simulink model "c6711dsktest"  (Simulink 6.0)
settings: Solver=FixedStepDiscrete  SolverMode=SingleTasking  StartTime=0.0  StopTime=inf  RelTol=1e-3
libraries: c6711dsklib x3, c6000tgtpreflib x1, dspsrcs4 x1
settings Model: Creator=tjones  LastModifiedBy=thartley  ExtModeTrigMode=oneshot  ExtModeArmWhenConnect=off  ProdHWDeviceType=TI C6000
settings DataIOCC: LimitDataPoints=off  SaveOutput=off  SaveTime=off  SignalLoggingName=sigsOut
settings OptimizationCC: BlockReduction=off  BooleanDataType=off  InlineParams=on  LocalBlockOutputs=off  RollThreshold=2
settings DebuggingCC: AlgebraicLoopMsg=error  CheckExecutionContextPreStartOutputMsg=on  CheckExecutionContextRuntimeOutputMsg=on  SolverPrmCheckMsg=none
settings HardwareCC: ProdBitPerLong=40  ProdEndianess=LittleEndian  ProdHWDeviceType=TI C6000
settings ModelReferenceCC: UpdateModelReferenceTargets=IfOutOfDate
settings RTWCC: SystemTargetFile=ti_c6000.tlc  TemplateMakefile=ti_c6000.tmf  ProcessScript=ti_c6000_make_rtw_hook
settings CodeAppCC: PrefixModelToSubsysFcnNames=off
settings STFCustomTargetCC: TargetFcnLib=ansi_tfl_tmw.mat  MatFileLogging=on  LifeSpan=inf  SystemTargetFile=ti_c6000.tlc  ActivateCallback=c6000_callback('ActivateCallback',hSrc,hDlg);
settings GRTTargetCC: ModelReferenceCompliant=off  LifeSpan=inf
settings CustomProperty: DataType=RTWOptions_EnumType_S__A_matlab_toolbox_rtw_targets_tic6000_tic6000_ti_c6000_BoardType  Value=C6711DSK
settings EnumStrPairs: String=C6416DSK
settings SFSimCC: SFSimApplyToAllLibs=on  SFSimBuildMode=Incremental

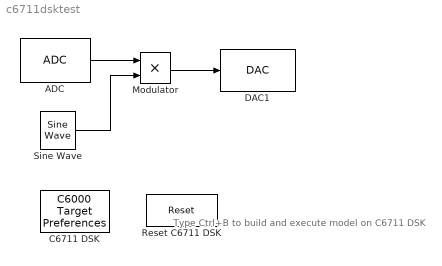
== system c6711dsktest ==
  note: Type Ctrl+B to build
      | and execute model
      | on C6711 DSK
  ADC : c6711dsklib/ADC  ADCsource=Line In  MicGain=off  OutputDataType=Double  Scaling=Normalize  SourceGain=0.0  FrameSize=256
  C6711 DSK : c6000tgtpreflib/C6000 Target Preferences
  DAC1 : c6711dsklib/DAC  Scaling=Normalize  DacAtten=0.0  OverflowMode=Saturate
  Modulator : Product  SaturateOnIntegerOverflow=on  InputSameDT=on
  Reset C6711 DSK : c6711dsklib/Reset
  Sine Wave : dspsrcs4/Sine Wave  Amplitude=1  Frequency=2000  Phase=0  SampleMode=Discrete  OutComplex=Real  CompMethod=Differential  TableSize=Speed  SampleTime=1/8000  SamplesPerFrame=256  dataType=double  wordLen=16  udDataType=sfix(16)  fracBitsMode=Best precision  numFracBits=14  ResetState=Restart at time zero
  wires:
  ADC/1 -> Modulator/1
  Modulator/1 -> DAC1/1
  Sine Wave/1 -> Modulator/2
